simulink model "pendulo_sim"  (R2019b)
settings: Solver=ode4  StartTime=0.0  StopTime=t_sim  FixedStep=0.01  RelTol=1e-3
values from neighbouring files (symbols this model uses):
  alpha_dot_0 = 2*pi/4    (= 1.57079632679)    [pendulo.m]    (also in pendulo_en_movimiento.m)
  alpha_dot_dot_0 = 2*pi/4    (= 1.57079632679)    [pendulo.m]    (also in pendulo_en_movimiento.m)
  B = 2    [pendulo.m]    (also in pendulo_en_movimiento.m = Bs(1))
  c = cos(theta_0)    [pendulo_en_movimiento.m]
  g = 9.8    [pendulo.m]    (also in pendulo_en_movimiento.m)
  J = m*l^2    (= 3)    [pendulo.m]    (also in pendulo_en_movimiento.m = m*l^2)
  l = 1    [pendulo.m]    (also in pendulo_en_movimiento.m = l_s(1))
  m = 3    [pendulo.m]    (also in pendulo_en_movimiento.m = ms(1))
settings Model: Creator=5danalfaro  LastModifiedBy=5danalfaro

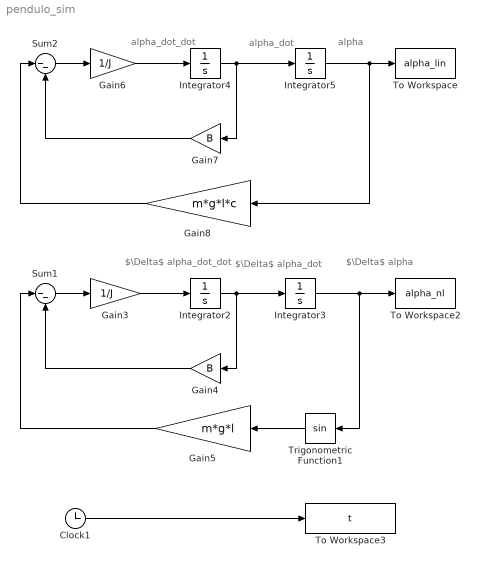
== system pendulo_sim ==
  note: alpha
  note: alpha_dot
  note: $\Delta$ alpha_dot
  note: $\Delta$ alpha_dot_dot
  note: alpha_dot_dot
  note: $\Delta$ alpha
  Clock1 : Clock
  Gain3 : Gain  Gain=1/J
  Gain4 : Gain  Gain=B
  Gain5 : Gain  Gain=m*g*l
  Gain6 : Gain  Gain=1/J
  Gain7 : Gain  Gain=B
  Gain8 : Gain  Gain=m*g*l*c
  Integrator2 : Integrator  InitialCondition=alpha_dot_dot_0
  Integrator3 : Integrator  InitialCondition=alpha_dot_0
  Integrator4 : Integrator  InitialCondition=alpha_dot_dot_0
  Integrator5 : Integrator  InitialCondition=alpha_dot_0
  Sum1 : Sum  Inputs=|--
  Sum2 : Sum  Inputs=|--
  To Workspace : ToWorkspace  VariableName=alpha_lin  SampleTime=-1
  To Workspace2 : ToWorkspace  VariableName=alpha_nl  SampleTime=-1
  To Workspace3 : ToWorkspace  VariableName=t  SampleTime=-1
  Trigonometric Function1 : Trigonometry
  wires:
  Integrator5/1 -> Gain8/1, To Workspace/1
  Trigonometric Function1/1 -> Gain5/1
  Sum2/1 -> Gain6/1
  Integrator2/1 -> Gain4/1, Integrator3/1
  Gain6/1 -> Integrator4/1
  Integrator3/1 -> Trigonometric Function1/1, To Workspace2/1
  Gain5/1 -> Sum1/1
  Gain3/1 -> Integrator2/1
  Clock1/1 -> To Workspace3/1
  Gain4/1 -> Sum1/2
  Gain8/1 -> Sum2/1
  Gain7/1 -> Sum2/2
  Sum1/1 -> Gain3/1
  Integrator4/1 -> Gain7/1, Integrator5/1
